simulink model "DC_motor"  (R2024a)
settings: Solver=ode45  StartTime=0.0  StopTime=0.4  RelTol=1e-4
values from neighbouring files (symbols this model uses):
  B = 0.1    [set_DC_motor_param.m]
  J = .00252    (= 0.00252)    [set_DC_motor_param.m]
  K = Te_rated/Ia_rated    (= 0.424752712124)    [set_DC_motor_param.m]
  La = 1.7e-3    (= 0.0017)    [set_DC_motor_param.m]
  Ra = 0.26    [set_DC_motor_param.m]
settings Model: Creator=CDSL-2  LastModifiedBy=CDSL-2

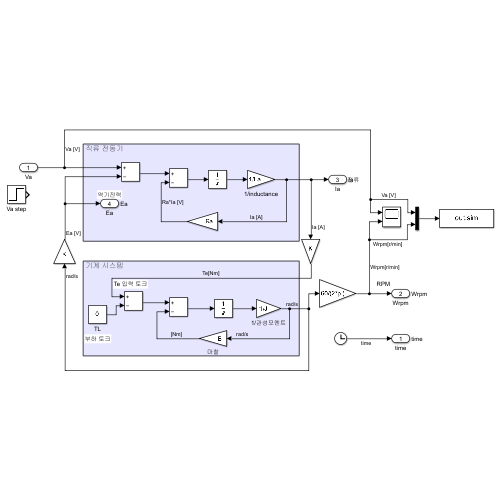
[thumbnail: Simulink's stored preview of the top-level diagram]
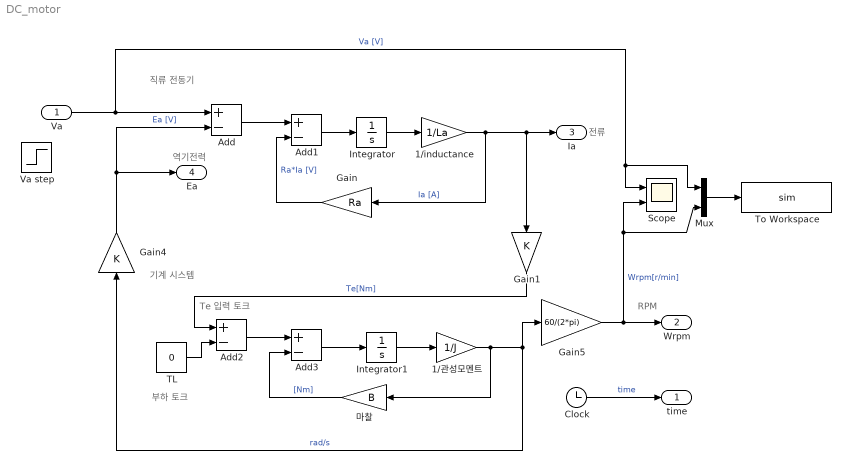
== system DC_motor ==
  note: Te 입력 토크
  note: RPM
  note: 전류
  note: 역기전력
  note: 부하 토크
  note: 기계 시스템
  note: 직류 전동기
  Va : Inport
  1/inductance : Gain  Gain=1/La
  1/관성모멘트 : Gain  Gain=1/J
  Add{,1..3} (4 alike) : Sum  Inputs=+-
  Clock : Clock
  Gain : Gain  Gain=Ra
  Gain1 : Gain  Gain=K
  Gain4 : Gain  Gain=K
  Gain5 : Gain  Gain=60/(2*pi)
  Integrator : Integrator
  Integrator1 : Integrator
  Mux : Mux  Inputs=2
  Scope : Scope  NumInputPorts=2
  TL : Constant  Value=0
  To Workspace : ToWorkspace  VariableName=sim  SaveFormat=Timeseries  SampleTime=-1
  Va step : Step  Time=0.05  After=140  SampleTime=0
  마찰 : Gain  Gain=B
  time : Outport  SignalName=time  Unit=s
  Wrpm : Outport  Port=2  SignalName=Wrpm  Unit=rpm
  Ia : Outport  Port=3  SignalName=Ia  Unit=A
  Ea : Outport  Port=4  SignalName=Ea  Unit=V
  wires:
  Add/1 -> Add1/1
  Add1/1 -> Integrator/1
  Gain/1 -> Add1/2  "Ra*Ia [V]"
  Integrator/1 -> 1/inductance/1
  Gain1/1 -> Add2/1  "Te[Nm]"
  TL/1 -> Add2/2
  Add2/1 -> Add3/1
  Add3/1 -> Integrator1/1
  Integrator1/1 -> 1/관성모멘트/1
  1/관성모멘트/1 -> Gain4/1, Gain5/1, 마찰/1  "rad/s"
  마찰/1 -> Add3/2  "[Nm]"
  Gain4/1 -> Ea/1, Add/2  "Ea [V]"
  Clock/1 -> time/1  "time"
  1/inductance/1 -> Ia/1, Gain1/1, Gain/1  "Ia [A]"
  Gain5/1 -> Scope/2, Mux/2, Wrpm/1  "Wrpm[r/min]"
  Va/1 -> Mux/1, Scope/1, Add/1  "Va [V]"
  Mux/1 -> To Workspace/1
